simulink library "ccsllib"  (R2017a)
settings: Solver=VariableStepAuto  StartTime=0.0  StopTime=10.0  RelTol=1e-3
libraries: simulink x1
settings Model: Creator=Li  LastModifiedBy=Li

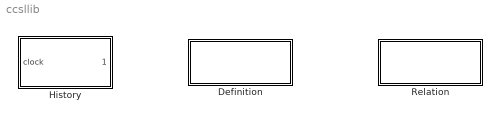
== system ccsllib ==
  Definition : Subsystem
      settings: OpenFcn=ccsldef
  History : Subsystem
      mask DialogControl Control2 Prompt: history
  Relation : Subsystem
      settings: OpenFcn=ccslrel

== system ccsllib/Definition ==

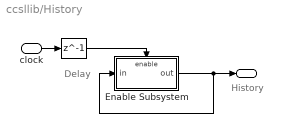
== system ccsllib/History ==
  note: History
  note: Delay
  clock : Inport
  " " : Delay  DelayLength=1  InitialCondition=0
  Enable Subsystem : Subsystem  TreatAsAtomicUnit=on
  " " : Outport
  wires:
  Enable Subsystem/1(out) -> Enable Subsystem/1("in "), " "/1
  " "/1 -> Enable Subsystem/Enable
  clock/1 -> " "/1

== system ccsllib/Relation ==

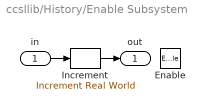
== system ccsllib/History/Enable Subsystem ==
  "in " : Inport
  Enable : EnablePort
  "Increment " : simulink/Additional Math & Discrete/Additional Math: Increment - Decrement/Increment Real World
      settings: SourceProductName=Simulink  SourceProductBaseCode=SL
  out : Outport
  wires:
  "Increment "/1 -> out/1
  "in "/1 -> "Increment "/1
